simulink model "FMLibrary_v2_progress"  (R2016b)
settings: Solver=VariableStepAuto  StartTime=0.0  StopTime=10.0  RelTol=1e-3
undefined symbols (not defined in the file or in its folder): Lb, Lf, Lu, RobotStruct, sampleTime
libraries: simulink x24, FM_Library x10, VariousBlocksLibrary x10, FMLibrary_v2 x2, simulink_extras x2
(part 1 of 3)
settings Model: Creator=niekbeckers  LastModifiedBy=niekbeckers

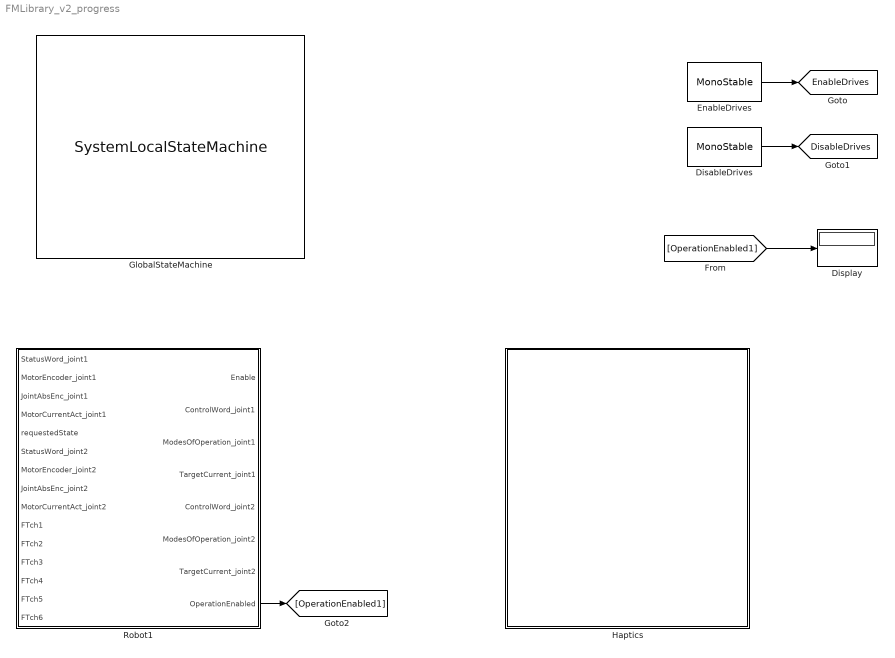
== system FMLibrary_v2_progress ==
  DisableDrives : FM_Library/MonoStable  Value=0  OutMin=[]  OutMax=[]  OutDataTypeStr=Inherit: Inherit from 'Constant value'
  Display : Display
  EnableDrives : FM_Library/MonoStable  Value=0  OutMin=[]  OutMax=[]  OutDataTypeStr=Inherit: Inherit from 'Constant value'
  GlobalStateMachine : FMLibrary_v2/StateMachineLocal/SystemLocalStateMachine
  Haptics : Subsystem
  Robot1 : Subsystem
  tag scope: DisableDrives=global, EnableDrives=global
  wires:
  DisableDrives/1 -> [DisableDrives]
  EnableDrives/1 -> [EnableDrives]
  Robot1/8(OperationEnabled) -> [OperationEnabled1]
  [OperationEnabled1] -> Display/1

== system FMLibrary_v2_progress/Haptics ==
  Bus Selector : BusSelector  OutputSignals=xOpSpace.x,xOpSpace.xdot
  tag scope: x_ref=global, xddot_ref=global, xdot_ref=global
  wires:
  [BusRobot1] -> Bus Selector/1

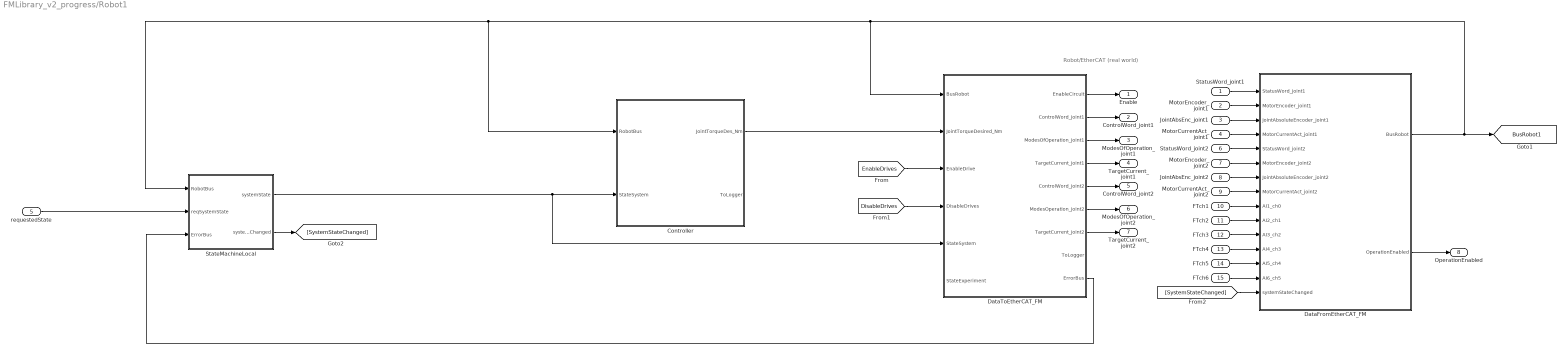
== system FMLibrary_v2_progress/Robot1 ==
  note: Robot/EtherCAT (real world)
  StatusWord_joint1 : Inport
  MotorEncoder_joint1 : Inport  Port=2
  JointAbsEnc_joint1 : Inport  Port=3
  MotorCurrentAct_joint1 : Inport  Port=4
  requestedState : Inport  Port=5
  StatusWord_joint2 : Inport  Port=6
  MotorEncoder_joint2 : Inport  Port=7
  JointAbsEnc_joint2 : Inport  Port=8
  MotorCurrentAct_joint2 : Inport  Port=9
  FTch1 : Inport  Port=10
  FTch2 : Inport  Port=11
  FTch3 : Inport  Port=12
  FTch4 : Inport  Port=13
  FTch5 : Inport  Port=14
  FTch6 : Inport  Port=15
  Controller : Subsystem  AncestorBlock=FMLibrary_v2/Controller
  DataFromEtherCAT_FM : Subsystem  AncestorBlock=FMLibrary_v2/DataFromEtherCAT_FM
  DataToEtherCAT_FM : Subsystem  AncestorBlock=FMLibrary_v2/DataToEtherCAT_FM
  StateMachineLocal : Subsystem  AncestorBlock=FMLibrary_v2/StateMachineLocal
  Enable : Outport
  ControlWord_joint1 : Outport  Port=2
  ModesOfOperation_joint1 : Outport  Port=3
  TargetCurrent_joint1 : Outport  Port=4
  ControlWord_joint2 : Outport  Port=5
  ModesOfOperation_joint2 : Outport  Port=6
  TargetCurrent_joint2 : Outport  Port=7
  OperationEnabled : Outport  Port=8
  tag scope: BusRobot1=global
  wires:
  DataFromEtherCAT_FM/2(OperationEnabled) -> OperationEnabled/1
  FTch3/1 -> DataFromEtherCAT_FM/11(AI3_ch2)
  FTch4/1 -> DataFromEtherCAT_FM/12(AI4_ch3)
  FTch6/1 -> DataFromEtherCAT_FM/14(AI6_ch5)
  StatusWord_joint2/1 -> DataFromEtherCAT_FM/5(StatusWord_joint2)
  StatusWord_joint1/1 -> DataFromEtherCAT_FM/1(StatusWord_joint1)
  DataToEtherCAT_FM/6(ModesOperation_joint2) -> ModesOfOperation_joint2/1
  DataToEtherCAT_FM/5(ControlWord_joint2) -> ControlWord_joint2/1
  MotorEncoder_joint1/1 -> DataFromEtherCAT_FM/2(MotorEncoder_joint1)
  JointAbsEnc_joint2/1 -> DataFromEtherCAT_FM/7("JointAbsoluteEncoder_joint2 ")
  FTch5/1 -> DataFromEtherCAT_FM/13(AI5_ch4)
  DataToEtherCAT_FM/4(TargetCurrent_joint1) -> TargetCurrent_joint1/1
  MotorCurrentAct_joint2/1 -> DataFromEtherCAT_FM/8(MotorCurrentAct_joint2)
  [EnableDrives] -> DataToEtherCAT_FM/3(EnableDrive)
  [DisableDrives] -> DataToEtherCAT_FM/4(DisableDrives)
  Controller/1(JointTorqueDes_Nm) -> DataToEtherCAT_FM/2(JointTorqueDesired_Nm)
  requestedState/1 -> StateMachineLocal/2(reqSystemState)
  DataFromEtherCAT_FM/1(BusRobot) -> [BusRobot1], DataToEtherCAT_FM/1(BusRobot), Controller/1(RobotBus), StateMachineLocal/1(RobotBus)
  DataToEtherCAT_FM/9(ErrorBus) -> StateMachineLocal/3(ErrorBus)
  [SystemStateChanged] -> DataFromEtherCAT_FM/15(systemStateChanged)
  StateMachineLocal/2(systemStateChanged) -> [SystemStateChanged]
  DataToEtherCAT_FM/2(ControlWord_joint1) -> ControlWord_joint1/1
  StateMachineLocal/1(systemState) -> DataToEtherCAT_FM/5(StateSystem), Controller/2(StateSystem)
  FTch1/1 -> DataFromEtherCAT_FM/9(AI1_ch0)
  DataToEtherCAT_FM/1(EnableCircuit) -> Enable/1
  DataToEtherCAT_FM/3(ModesOfOperation_joint1) -> ModesOfOperation_joint1/1
  JointAbsEnc_joint1/1 -> DataFromEtherCAT_FM/3(JointAbsoluteEncoder_joint1)
  MotorEncoder_joint2/1 -> DataFromEtherCAT_FM/6(MotorEncoder_joint2)
  MotorCurrentAct_joint1/1 -> DataFromEtherCAT_FM/4(MotorCurrentAct_joint1)
  FTch2/1 -> DataFromEtherCAT_FM/10(AI2_ch1)
  DataToEtherCAT_FM/7(TargetCurrent_joint2) -> TargetCurrent_joint2/1

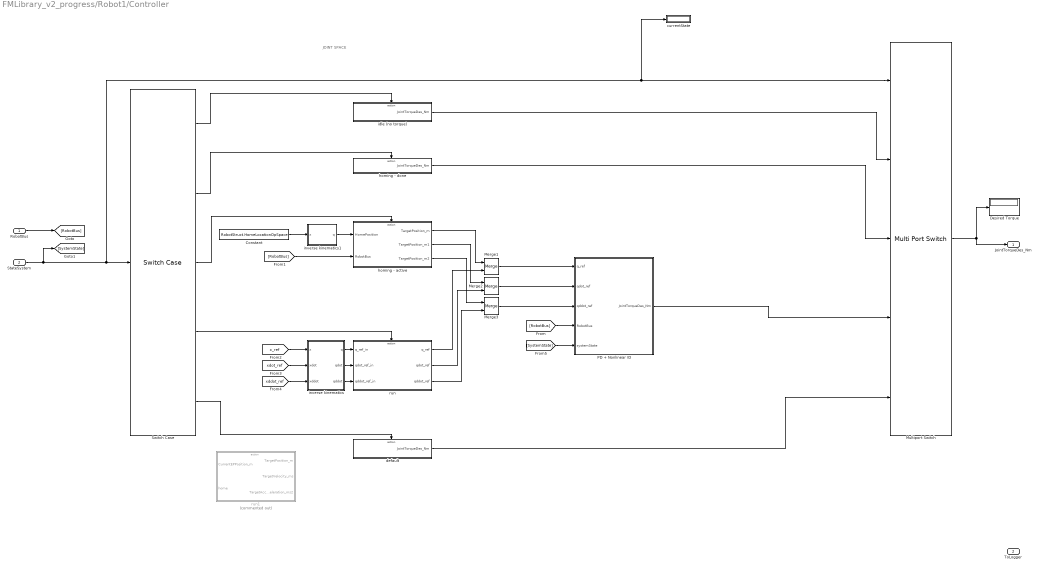
== system FMLibrary_v2_progress/Robot1/Controller ==
  note: JOINT SPACE
  RobotBus : Inport
  StateSystem : Inport  Port=2
  Constant : Constant  Value=RobotStruct.HomeLocationOpSpace
  Desired Torque : Display
  Merge1 : Merge  InitialOutput=[0;0]
  Merge2 : Merge  InitialOutput=[0;0]
  Merge3 : Merge  InitialOutput=[0;0]
  Multiport Switch : MultiPortSwitch  DataPortOrder=Specify indices  Inputs=4  DataPortIndices={[0,1,2,201,299,301],[399],[302,4]}  DataPortForDefault=Additional data port
  PD + Nonlinear ID : Subsystem
  Switch Case : SwitchCase  CaseConditions={[0,1,2,201,299,301],[399],[302],[4]}
  currentState : Display
  default : Subsystem  TreatAsAtomicUnit=on
  homing - active : Subsystem
  homing - done : Subsystem  TreatAsAtomicUnit=on
  idle (no torque) : Subsystem  TreatAsAtomicUnit=on
  inverse kinematics : MATLAB Function  TreatAsAtomicUnit=on
  inverse kinematics1 : MATLAB Function  TreatAsAtomicUnit=on
  run : Subsystem
  run1 : Subsystem  Commented=on
  JointTorqueDes_Nm : Outport
  ToLogger : Outport  Port=2
  wires:
  homing - active/3(TargetPosition_m2) -> Merge3/1
  homing - active/2(TargetPosition_m1) -> Merge2/1
  run/3(qddot_ref) -> Merge3/2
  run/2(qdot_ref) -> Merge2/2
  StateSystem/1 -> [SystemState], Switch Case/1, currentState/1, Multiport Switch/1
  run/1(q_ref) -> Merge1/2
  homing - active/1(TargetPosition_m) -> Merge1/1
  Switch Case/4 -> run/Action
  Multiport Switch/1 -> JointTorqueDes_Nm/1, Desired Torque/1
  Switch Case/5 -> default/Action
  default/1(JointTorqueDes_Nm) -> Multiport Switch/5
  Switch Case/1 -> idle (no torque)/Action
  Switch Case/3 -> homing - active/Action
  Switch Case/2 -> homing - done/Action
  idle (no torque)/1(JointTorqueDes_Nm) -> Multiport Switch/2
  homing - done/1(JointTorqueDes_Nm) -> Multiport Switch/3
  Merge1/1 -> PD + Nonlinear ID/1(q_ref)
  Merge2/1 -> PD + Nonlinear ID/2(qdot_ref)
  Merge3/1 -> PD + Nonlinear ID/3(qddot_ref)
  PD + Nonlinear ID/1(JointTorqueDes_Nm) -> Multiport Switch/4
  RobotBus/1 -> [RobotBus]
  [RobotBus] -> PD + Nonlinear ID/4(RobotBus)
  [RobotBus] -> homing - active/2(RobotBus)
  Constant/1 -> inverse kinematics1/1(x)
  inverse kinematics/1(q) -> run/1(q_ref_in)
  inverse kinematics/2(qdot) -> run/2(qdot_ref_in)
  inverse kinematics/3(qddot) -> run/3(qddot_ref_in)
  [x_ref] -> inverse kinematics/1(x)
  [xdot_ref] -> inverse kinematics/2(xdot)
  [xddot_ref] -> inverse kinematics/3(xddot)
  inverse kinematics1/1(q) -> homing - active/1(HomePosition)
  [SystemState] -> PD + Nonlinear ID/5(systemState)

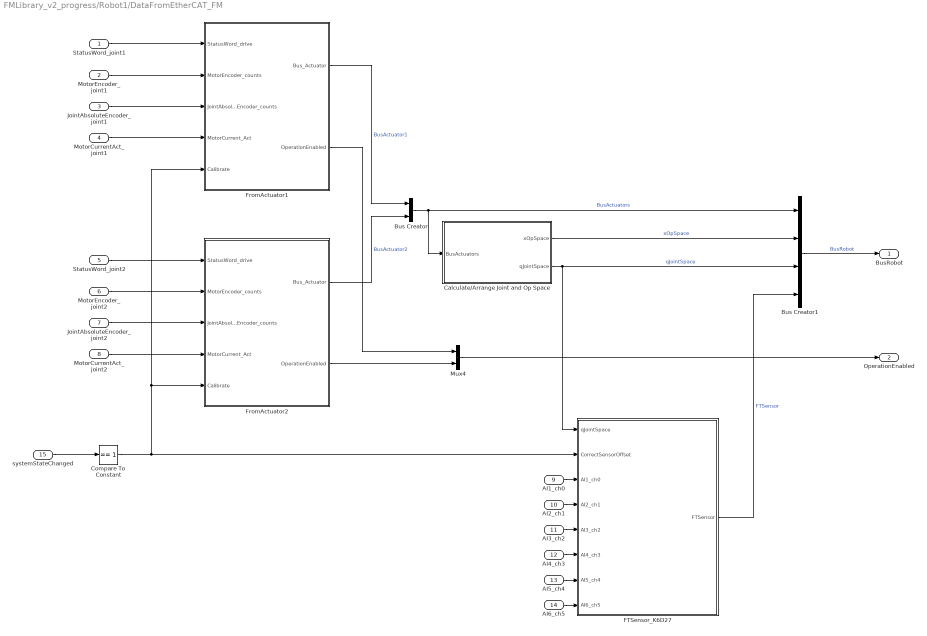
== system FMLibrary_v2_progress/Robot1/DataFromEtherCAT_FM ==
  StatusWord_joint1 : Inport
  MotorEncoder_joint1 : Inport  Port=2
  JointAbsoluteEncoder_joint1 : Inport  Port=3
  MotorCurrentAct_joint1 : Inport  Port=4
  StatusWord_joint2 : Inport  Port=5
  MotorEncoder_joint2 : Inport  Port=6
  "JointAbsoluteEncoder_joint2 " : Inport  Port=7
  MotorCurrentAct_joint2 : Inport  Port=8
  AI1_ch0 : Inport  Port=9  OutDataTypeStr=int16
  AI2_ch1 : Inport  Port=10  OutDataTypeStr=int16
  AI3_ch2 : Inport  Port=11  OutDataTypeStr=int16
  AI4_ch3 : Inport  Port=12  OutDataTypeStr=int16
  AI5_ch4 : Inport  Port=13  OutDataTypeStr=int16
  AI6_ch5 : Inport  Port=14  OutDataTypeStr=int16
  systemStateChanged : Inport  Port=15
  Bus Creator : BusCreator  Inputs=2
  Bus Creator1 : BusCreator  Inputs=4
  Calculate/Arrange Joint and Op Space : Subsystem
  Compare To Constant : simulink/Logic and Bit Operations/Compare To Constant  relop===  const=1  OutDataTypeStr=boolean
  FTSensor_K6D27 : Subsystem  mask{FTSensorStruct=RobotStruct.FTSensor}
      mask prompts: FTSensorStruct "Struct for force torque sensor"
  FromActuator1 : Subsystem  AncestorBlock=FMLibrary_v2/FromActuator1  mask{ActuatorStruct=RobotStruct.ActuatorStruct}
      mask prompts: ActuatorStruct "Actuator Struct"
  FromActuator2 : Subsystem  AncestorBlock=FMLibrary_v2/FromActuator1  mask{ActuatorStruct=RobotStruct.ActuatorStruct}
      mask prompts: ActuatorStruct "Actuator Struct"
  Mux4 : Mux  Inputs=2
  BusRobot : Outport
  OperationEnabled : Outport  Port=2
  wires:
  Compare To Constant/1 -> FTSensor_K6D27/2(CorrectSensorOffset), FromActuator1/5(Calibrate), FromActuator2/5(Calibrate)
  FTSensor_K6D27/1(FTSensor) -> Bus Creator1/4  "FTSensor"
  AI6_ch5/1 -> FTSensor_K6D27/8(AI6_ch5)
  AI5_ch4/1 -> FTSensor_K6D27/7(AI5_ch4)
  AI4_ch3/1 -> FTSensor_K6D27/6(AI4_ch3)
  AI3_ch2/1 -> FTSensor_K6D27/5(AI3_ch2)
  AI2_ch1/1 -> FTSensor_K6D27/4(AI2_ch1)
  AI1_ch0/1 -> FTSensor_K6D27/3(AI1_ch0)
  systemStateChanged/1 -> Compare To Constant/1
  Calculate/Arrange Joint and Op Space/2(qJointSpace) -> Bus Creator1/3, FTSensor_K6D27/1(qJointSpace)  "qJointSpace"
  Calculate/Arrange Joint and Op Space/1(xOpSpace) -> Bus Creator1/2  "xOpSpace"
  Bus Creator1/1 -> BusRobot/1  "BusRobot"
  Bus Creator/1 -> Bus Creator1/1, Calculate/Arrange Joint and Op Space/1(BusActuators)  "BusActuators"
  MotorCurrentAct_joint2/1 -> FromActuator2/4(MotorCurrent_Act)
  "JointAbsoluteEncoder_joint2 "/1 -> FromActuator2/3(JointAbsoluteEncoder_counts)
  StatusWord_joint2/1 -> FromActuator2/1(StatusWord_drive)
  MotorEncoder_joint2/1 -> FromActuator2/2(MotorEncoder_counts)
  MotorCurrentAct_joint1/1 -> FromActuator1/4(MotorCurrent_Act)
  JointAbsoluteEncoder_joint1/1 -> FromActuator1/3(JointAbsoluteEncoder_counts)
  StatusWord_joint1/1 -> FromActuator1/1(StatusWord_drive)
  MotorEncoder_joint1/1 -> FromActuator1/2(MotorEncoder_counts)
  FromActuator2/2(OperationEnabled) -> Mux4/2
  Mux4/1 -> OperationEnabled/1
  FromActuator1/2(OperationEnabled) -> Mux4/1
  FromActuator2/1(Bus_Actuator) -> Bus Creator/2  "BusActuator2"
  FromActuator1/1(Bus_Actuator) -> Bus Creator/1  "BusActuator1"

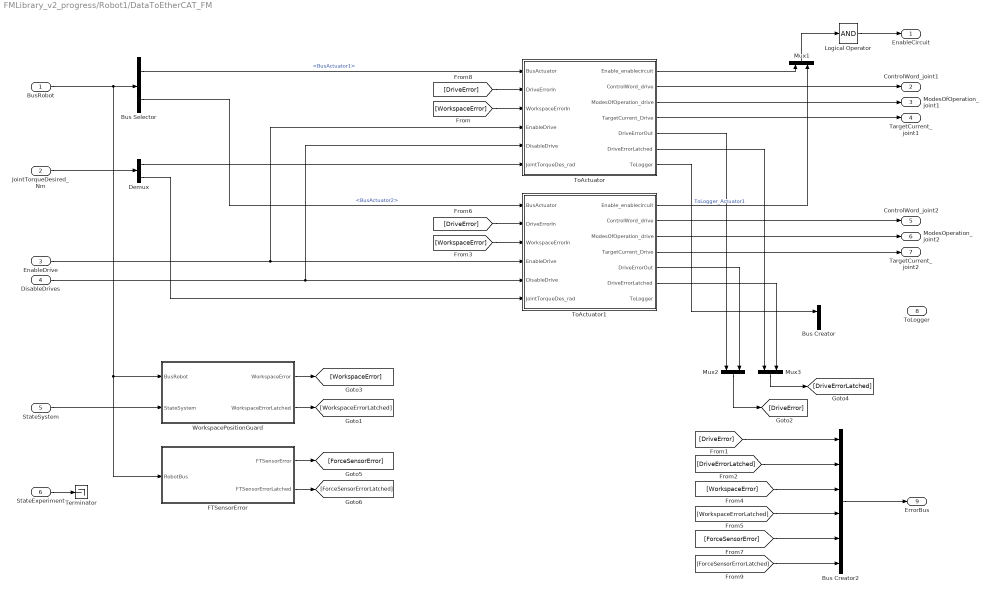
== system FMLibrary_v2_progress/Robot1/DataToEtherCAT_FM ==
  BusRobot : Inport
  JointTorqueDesired_Nm : Inport  Port=2
  EnableDrive : Inport  Port=3
  DisableDrives : Inport  Port=4
  StateSystem : Inport  Port=5
  StateExperiment : Inport  Port=6
  Bus Creator : BusCreator  Inputs=2
  Bus Creator2 : BusCreator  Inputs=6
  Bus Selector : BusSelector  OutputSignals=BusActuators.BusActuator1,BusActuators.BusActuator2
  Demux : Demux  Outputs=2
  FTSensorError : Subsystem
  Logical Operator : Logic  Inputs=1  AllPortsSameDT=off  OutDataTypeStr=boolean
  Mux1 : Mux  Inputs=2
  Mux2 : Mux  Inputs=2
  Mux3 : Mux  Inputs=2
  Terminator : Terminator
  ToActuator : Subsystem  AncestorBlock=FMLibrary_v2/ToActuator  mask{ActuatorStruct=RobotStruct.Actuator1}
      mask prompts: ActuatorStruct "Actuator Struct"
  ToActuator1 : Subsystem  AncestorBlock=FMLibrary_v2/ToActuator  mask{ActuatorStruct=RobotStruct.Actuator1}
      mask prompts: ActuatorStruct "Actuator Struct"
  WorkspacePositionGuard : Subsystem
  EnableCircuit : Outport
  ControlWord_joint1 : Outport  Port=2
  ModesOfOperation_joint1 : Outport  Port=3
  TargetCurrent_joint1 : Outport  Port=4
  ControlWord_joint2 : Outport  Port=5
  ModesOperation_joint2 : Outport  Port=6
  TargetCurrent_joint2 : Outport  Port=7
  ToLogger : Outport  Port=8
  ErrorBus : Outport  Port=9
  wires:
  StateExperiment/1 -> Terminator/1
  [ForceSensorErrorLatched] -> Bus Creator2/6
  [ForceSensorError] -> Bus Creator2/5
  FTSensorError/2(FTSensorErrorLatched) -> [ForceSensorErrorLatched]
  FTSensorError/1(FTSensorError) -> [ForceSensorError]
  StateSystem/1 -> WorkspacePositionGuard/2(StateSystem)
  [WorkspaceErrorLatched] -> Bus Creator2/4
  [WorkspaceError] -> Bus Creator2/3
  [DriveErrorLatched] -> Bus Creator2/2
  [DriveError] -> Bus Creator2/1
  Bus Creator2/1 -> ErrorBus/1
  Mux3/1 -> [DriveErrorLatched]
  [WorkspaceError] -> ToActuator1/3(WorkspaceErrorIn)
  [DriveError] -> ToActuator1/2(DriveErrorIn)
  EnableDrive/1 -> ToActuator1/4(EnableDrive), ToActuator/4(EnableDrive)
  DisableDrives/1 -> ToActuator1/5(DisableDrive), ToActuator/5(DisableDrive)
  [WorkspaceError] -> ToActuator/3(WorkspaceErrorIn)
  WorkspacePositionGuard/1(WorkspaceError) -> [WorkspaceError]
  WorkspacePositionGuard/2(WorkspaceErrorLatched) -> [WorkspaceErrorLatched]
  Bus Selector/1 -> ToActuator/1(BusActuator)  "<BusActuator1>"
  Bus Selector/2 -> ToActuator1/1(BusActuator)  "<BusActuator2>"
  BusRobot/1 -> Bus Selector/1, WorkspacePositionGuard/1(BusRobot), FTSensorError/1(RobotBus)
  Demux/1 -> ToActuator/6(JointTorqueDes_rad)
  JointTorqueDesired_Nm/1 -> Demux/1
  Demux/2 -> ToActuator1/6(JointTorqueDes_rad)
  Logical Operator/1 -> EnableCircuit/1
  ToActuator1/3(ModesOfOperation_drive) -> ModesOperation_joint2/1
  ToActuator1/4(TargetCurrent_Drive) -> TargetCurrent_joint2/1
  ToActuator/4(TargetCurrent_Drive) -> TargetCurrent_joint1/1
  ToActuator1/2(ControlWord_drive) -> ControlWord_joint2/1
  ToActuator/3(ModesOfOperation_drive) -> ModesOfOperation_joint1/1
  ToActuator/2(ControlWord_drive) -> ControlWord_joint1/1
  ToActuator1/1(Enable_enablecircuit) -> Mux1/2
  ToActuator/1(Enable_enablecircuit) -> Mux1/1
  Mux1/1 -> Logical Operator/1
  [DriveError] -> ToActuator/2(DriveErrorIn)
  ToActuator1/6(DriveErrorLatched) -> Mux3/2
  ToActuator/6(DriveErrorLatched) -> Mux3/1
  Mux2/1 -> [DriveError]
  ToActuator1/5(DriveErrorOut) -> Mux2/2
  ToActuator/5(DriveErrorOut) -> Mux2/1
  ToActuator/7(ToLogger) -> Bus Creator/1  "ToLogger_Actuator1"

== system FMLibrary_v2_progress/Robot1/StateMachineLocal ==
  note: Encode system state change - powers of 2 indicate which state change occurs.
  RobotBus : Inport
  reqSystemState : Inport  Port=2
  ErrorBus : Inport  Port=3
  Bus Selector : BusSelector  OutputSignals=xOpSpace.x,xOpSpace.xdot
  Constant : Constant  Value=RobotStruct.HomeLocationSize
  Constant1 : Constant  Value=RobotStruct.HomeLocationOpSpace
  Detect Change1 : simulink/Logic and Bit Operations/Detect Change  vinit=0  InputProcessing=Inherited  OutDataTypeStr=boolean
  Encode system state change : MATLAB Function  TreatAsAtomicUnit=on
  SystemLocalStateMachine : Stateflow chart  TreatAsAtomicUnit=on
  systemState : Outport
  systemStateChanged : Outport  Port=2
  wires:
  Bus Selector/2 -> SystemLocalStateMachine/4(xdot)  "<xdot>"
  Bus Selector/1 -> SystemLocalStateMachine/3(x)  "<x>"
  RobotBus/1 -> Bus Selector/1
  Constant1/1 -> SystemLocalStateMachine/5(HomePosition)
  Constant/1 -> SystemLocalStateMachine/6(homeLocationSize)
  Encode system state change/1(systemStateChanged) -> systemStateChanged/1
  Detect Change1/1 -> Encode system state change/1(stateChanged)
  ErrorBus/1 -> SystemLocalStateMachine/2(error)
  SystemLocalStateMachine/1(currentSystemState) -> Encode system state change/2(state), Detect Change1/1, systemState/1
  reqSystemState/1 -> SystemLocalStateMachine/1(reqSystemState)

== system FMLibrary_v2_progress/Robot1/Controller/PD + Nonlinear ID ==
  q_ref : Inport
  qdot_ref : Inport  Port=2
  qddot_ref : Inport  Port=3
  RobotBus : Inport  Port=4
  systemState : Inport  Port=5
  AFFC : Subsystem
  Bus Selector : BusSelector  OutputSignals=qJointSpace.q,qJointSpace.qdot
  DesiredTorque_PID : Display
  Gain : Gain
  Kd : Gain  Gain=0.1
  Kp : Gain  Gain=0.5
  Sum : Sum  Inputs=|+-
  Sum1 : Sum  Inputs=++|
  Sum2 : Sum  Inputs=|+-
  Sum3 : Sum  Inputs=|++
  p : Display
  JointTorqueDes_Nm : Outport
  wires:
  Bus Selector/2 -> Sum2/2  "<qdot>"
  Bus Selector/1 -> Sum/2  "<q>"
  q_ref/1 -> AFFC/1(q_ref), Sum/1
  Sum/1 -> Kp/1
  Sum3/1 -> AFFC/4(e), Sum1/2
  Kd/1 -> Sum3/2
  Kp/1 -> Sum3/1
  qdot_ref/1 -> AFFC/2(qdot_ref), Sum2/1
  Sum2/1 -> Kd/1
  Gain/1 -> Sum1/1
  Sum1/1 -> DesiredTorque_PID/1, JointTorqueDes_Nm/1
  RobotBus/1 -> Bus Selector/1
  qddot_ref/1 -> AFFC/3(qddot_ref)
  AFFC/1(p) -> p/1
  AFFC/2(tau_affc) -> Gain/1

== system FMLibrary_v2_progress/Robot1/Controller/default ==
  Action Port : ActionPort  InitializeStates=reset
  Constant3 : Constant  Value=[0;0]
  JointTorqueDes_Nm : Outport  InitialOutput=[0;0]
  wires:
  Constant3/1 -> JointTorqueDes_Nm/1

== system FMLibrary_v2_progress/Robot1/Controller/homing - active ==
  note: These blocks hold the first sample of the input
      | when the block is enabled (through the action port)
  HomePosition : Inport
  RobotBus : Inport  Port=2
  Action Port : ActionPort  InitializeStates=reset
  Bus Selector : BusSelector  OutputSignals=xOpSpace.x
  Constant1 : Constant
  Constant3 : Constant  Value=[0;0]
  Constant4 : Constant  Value=[0;0]
  Counter Free-Running : simulink/Sources/Counter Free-Running  NumBits=32  tsamp=-1
  CrossFade : VariousBlocksLibrary/Various/CrossFade
  Cycloid : VariousBlocksLibrary/Various/Cycloid
  Manual Switch : ManualSwitch  CurrentSetting=0
  Memory1 : Memory
  Rate Limiter : RateLimiter  RisingSlewLimit=0.2  FallingSlewLimit=-0.2  SampleTimeMode=inherited
  Switch : Switch  Threshold=1
  TargetPosition_m : Outport  InitialOutput=[0;0]
  TargetPosition_m1 : Outport  Port=2  InitialOutput=[0;0]
  TargetPosition_m2 : Outport  Port=3  InitialOutput=[0;0]
  wires:
  Constant4/1 -> TargetPosition_m2/1
  Constant3/1 -> TargetPosition_m1/1
  CrossFade/1 -> TargetPosition_m/1
  Manual Switch/1 -> CrossFade/1
  Memory1/1 -> Switch/1
  Counter Free-Running/1 -> Switch/2
  Switch/1 -> Manual Switch/1, Memory1/1
  Constant1/1 -> Rate Limiter/1
  Rate Limiter/1 -> Cycloid/1
  Cycloid/1 -> CrossFade/3
  HomePosition/1 -> CrossFade/2
  RobotBus/1 -> Bus Selector/1
  Bus Selector/1 -> Switch/3, Manual Switch/2  "<x>"

== system FMLibrary_v2_progress/Robot1/Controller/homing - done ==
  Action Port : ActionPort
  Constant : Constant  Value=[0;0]
  JointTorqueDes_Nm : Outport
  wires:
  Constant/1 -> JointTorqueDes_Nm/1

== system FMLibrary_v2_progress/Robot1/Controller/idle (no torque) ==
  Action Port : ActionPort  InitializeStates=reset
  Constant3 : Constant  Value=[0;0]
  JointTorqueDes_Nm : Outport
  wires:
  Constant3/1 -> JointTorqueDes_Nm/1

== system FMLibrary_v2_progress/Robot1/Controller/run ==
  q_ref_in : Inport
  qdot_ref_in : Inport  Port=2
  qddot_ref_in : Inport  Port=3
  Action Port : ActionPort  InitializeStates=reset
  q_ref : Outport
  qdot_ref : Outport  Port=2
  qddot_ref : Outport  Port=3
  wires:
  q_ref_in/1 -> q_ref/1
  qddot_ref_in/1 -> qddot_ref/1
  qdot_ref_in/1 -> qdot_ref/1

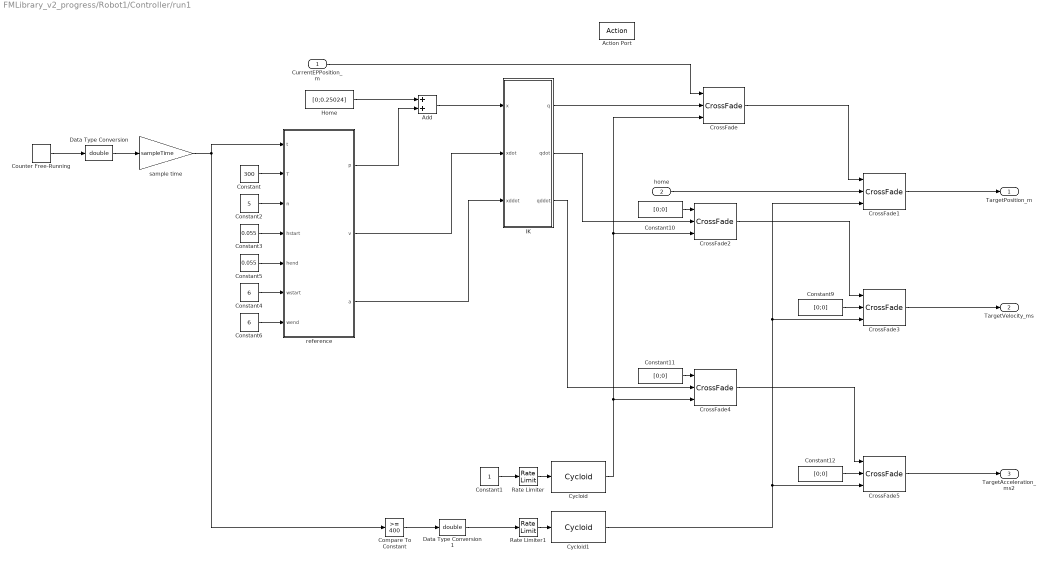
== system FMLibrary_v2_progress/Robot1/Controller/run1 ==
  CurrentEPPosition_m : Inport
  home : Inport  Port=2
  Action Port : ActionPort  InitializeStates=reset
  Add : Sum
  Compare To Constant : simulink/Logic and Bit Operations/Compare To Constant  relop=>=  const=400  OutDataTypeStr=boolean
  Constant : Constant  Value=300
  Constant1 : Constant
  Constant{9..12} (4 alike) : Constant  Value=[0;0]
  Constant2 : Constant  Value=5
  Constant3 : Constant  Value=0.055
  Constant4 : Constant  Value=6
  Constant5 : Constant  Value=0.055
  Constant6 : Constant  Value=6
  Counter Free-Running : simulink/Sources/Counter Free-Running  NumBits=32  tsamp=-1
  CrossFade{,1..5} (6 alike) : VariousBlocksLibrary/Various/CrossFade
  Cycloid : VariousBlocksLibrary/Various/Cycloid
  Cycloid1 : VariousBlocksLibrary/Various/Cycloid
  Data Type Conversion : DataTypeConversion  OutDataTypeStr=double
  Data Type Conversion1 : DataTypeConversion  OutDataTypeStr=double
  "Home " : Constant  Value=[0;0.25024]
  IK : MATLAB Function  TreatAsAtomicUnit=on
  Rate Limiter : RateLimiter  RisingSlewLimit=0.25  FallingSlewLimit=-0.15  SampleTimeMode=inherited
  Rate Limiter1 : RateLimiter  RisingSlewLimit=0.2  FallingSlewLimit=-0.2  SampleTimeMode=inherited
  reference : MATLAB Function  TreatAsAtomicUnit=on
  sample time : Gain  Gain=sampleTime
  TargetPosition_m : Outport
  TargetVelocity_ms : Outport  Port=2
  TargetAcceleration_ms2 : Outport  Port=3
  wires:
  Data Type Conversion1/1 -> Rate Limiter1/1
  IK/3(qddot) -> CrossFade4/2
  IK/1(q) -> CrossFade/2
  IK/2(qdot) -> CrossFade2/2
  "Home "/1 -> Add/1
  Add/1 -> IK/1(x)
  reference/1(p) -> Add/2
  reference/2(v) -> IK/2(xdot)
  reference/3(a) -> IK/3(xddot)
  Constant4/1 -> reference/6(wstart)
  Constant6/1 -> reference/7(wend)
  Constant3/1 -> reference/4(hstart)
  Constant5/1 -> reference/5(hend)
  Constant2/1 -> reference/3(n)
  Constant/1 -> reference/2(T)
  sample time/1 -> reference/1(t), Compare To Constant/1
  Counter Free-Running/1 -> Data Type Conversion/1
  Data Type Conversion/1 -> sample time/1
  CrossFade5/1 -> TargetAcceleration_ms2/1
  Constant11/1 -> CrossFade4/1
  Constant12/1 -> CrossFade5/2
  CrossFade4/1 -> CrossFade5/1
  Constant10/1 -> CrossFade2/1
  Constant9/1 -> CrossFade3/2
  CrossFade2/1 -> CrossFade3/1
  CrossFade3/1 -> TargetVelocity_ms/1
  Cycloid1/1 -> CrossFade1/3, CrossFade3/3, CrossFade5/3
  Rate Limiter1/1 -> Cycloid1/1
  Compare To Constant/1 -> Data Type Conversion1/1
  home/1 -> CrossFade1/2
  CrossFade/1 -> CrossFade1/1
  CrossFade1/1 -> TargetPosition_m/1
  CurrentEPPosition_m/1 -> CrossFade/1
  Rate Limiter/1 -> Cycloid/1
  Constant1/1 -> Rate Limiter/1
  Cycloid/1 -> CrossFade4/3, CrossFade/3, CrossFade2/3

== system FMLibrary_v2_progress/Robot1/DataFromEtherCAT_FM/Calculate//Arrange Joint and Op Space ==
  note: Here all angles of the parallel mechanism are calculated
      | based on the endpoint position, though this may still lead to incorrect
      | estimations of the internal angles (e.g. it is possible that on of the elbows
      | has gone through a singular position already). So perhaps I should also include
      | a different way of calculating the internal angles
  BusActuators : Inport
  Bus Creator1 : BusCreator  Inputs=3
  Bus Creator2 : BusCreator  Inputs=3
  Bus Selector : BusSelector  OutputSignals=BusActuator1.JointPosition_rad,BusActuator2.JointPosition_rad  OutputAsBus=on
  Bus Selector1 : BusSelector  OutputSignals=BusActuator1.JointVelocity_rads,BusActuator2.JointVelocity_rads  OutputAsBus=on
  Bus Selector2 : BusSelector  OutputSignals=BusActuator1.JointPosition_rad,BusActuator2.JointPosition_rad,BusActuator1.JointVelocity_rads,BusActuator2.JointVelocity_rads
  Ground : Ground
  IK all joints : MATLAB Function  TreatAsAtomicUnit=on
  Mux : Mux  Inputs=2
  Mux1 : Mux  Inputs=2
  Terminator1 : Terminator
  Terminator2 : Terminator
  forward kinematics : Subsystem
  xOpSpace : Outport
  qJointSpace : Outport  Port=2
  wires:
  IK all joints/1(q_all) -> Bus Creator2/3  "qall"
  Mux1/1 -> Bus Creator2/2  "qdot"
  Bus Selector2/4 -> Mux1/2  "<JointVelocity_rads>"
  Bus Selector2/3 -> Mux1/1  "<JointVelocity_rads>"
  Bus Selector2/2 -> Mux/2  "<JointPosition_rad>"
  Bus Selector2/1 -> Mux/1  "<JointPosition_rad>"
  Mux/1 -> Bus Creator2/1  "q"
  BusActuators/1 -> Bus Selector/1, Bus Selector2/1, Bus Selector1/1
  Bus Creator2/1 -> qJointSpace/1  "JointSpace"
  Ground/1 -> forward kinematics/3(JointAcceleration_rads2)
  Bus Selector1/1 -> forward kinematics/2(JointVelocity_rads)
  forward kinematics/4(J) -> Bus Creator1/3  "jacobian"
  Bus Creator1/1 -> xOpSpace/1  "OpSpace"
  forward kinematics/1(x) -> Bus Creator1/1, IK all joints/1(x)  "x"
  Bus Selector/1 -> forward kinematics/1(JointPosition_rad)
  forward kinematics/2(xdot) -> Bus Creator1/2  "xdot"
  forward kinematics/3(xddot) -> Terminator1/1
  forward kinematics/5(Jdot) -> Terminator2/1

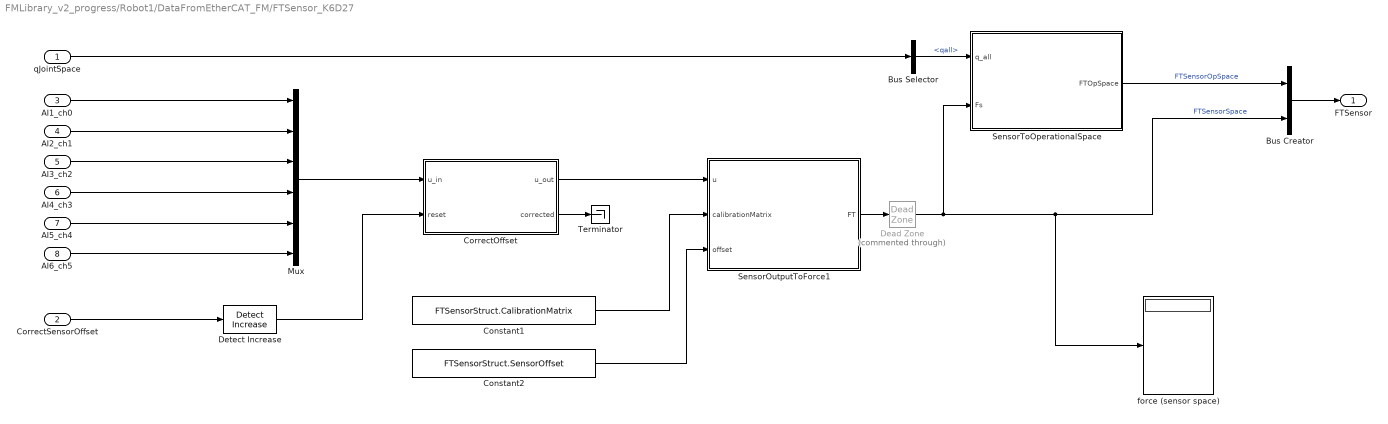
== system FMLibrary_v2_progress/Robot1/DataFromEtherCAT_FM/FTSensor_K6D27 ==
  qJointSpace : Inport
  CorrectSensorOffset : Inport  Port=2
  AI1_ch0 : Inport  Port=3  OutDataTypeStr=int16
  AI2_ch1 : Inport  Port=4  OutDataTypeStr=int16
  AI3_ch2 : Inport  Port=5  OutDataTypeStr=int16
  AI4_ch3 : Inport  Port=6  OutDataTypeStr=int16
  AI5_ch4 : Inport  Port=7  OutDataTypeStr=int16
  AI6_ch5 : Inport  Port=8  OutDataTypeStr=int16
  Bus Creator : BusCreator  Inputs=2
  Bus Selector : BusSelector  OutputSignals=qall
  Constant1 : Constant  Value=FTSensorStruct.CalibrationMatrix
  Constant2 : Constant  Value=FTSensorStruct.SensorOffset
  CorrectOffset : MATLAB Function  TreatAsAtomicUnit=on
  Dead Zone : DeadZone  Commented=through  LowerValue=-0.05  UpperValue=0.05  SaturateOnIntegerOverflow=on
  Detect Increase : simulink/Logic and Bit Operations/Detect Increase  vinit=0.0  InputProcessing=Inherited  OutDataTypeStr=boolean
  Mux : Mux  Inputs=6
  SensorOutputToForce1 : MATLAB Function  TreatAsAtomicUnit=on
  SensorToOperationalSpace : MATLAB Function  TreatAsAtomicUnit=on
  Terminator : Terminator
  force (sensor space) : Display
  FTSensor : Outport
  wires:
  SensorToOperationalSpace/1(FTOpSpace) -> Bus Creator/1  "FTSensorOpSpace"
  Bus Creator/1 -> FTSensor/1
  Constant2/1 -> SensorOutputToForce1/3(offset)
  Constant1/1 -> SensorOutputToForce1/2(calibrationMatrix)
  Dead Zone/1 -> SensorToOperationalSpace/2(Fs), force (sensor space)/1, Bus Creator/2  "FTSensorSpace"
  CorrectOffset/2(corrected) -> Terminator/1
  AI3_ch2/1 -> Mux/3
  AI4_ch3/1 -> Mux/4
  AI5_ch4/1 -> Mux/5
  AI6_ch5/1 -> Mux/6
  Bus Selector/1 -> SensorToOperationalSpace/1(q_all)  "<qall>"
  SensorOutputToForce1/1(FT) -> Dead Zone/1
  Detect Increase/1 -> CorrectOffset/2(reset)
  CorrectSensorOffset/1 -> Detect Increase/1
  Mux/1 -> CorrectOffset/1(u_in)
  CorrectOffset/1(u_out) -> SensorOutputToForce1/1(u)
  AI1_ch0/1 -> Mux/1
  AI2_ch1/1 -> Mux/2
  qJointSpace/1 -> Bus Selector/1

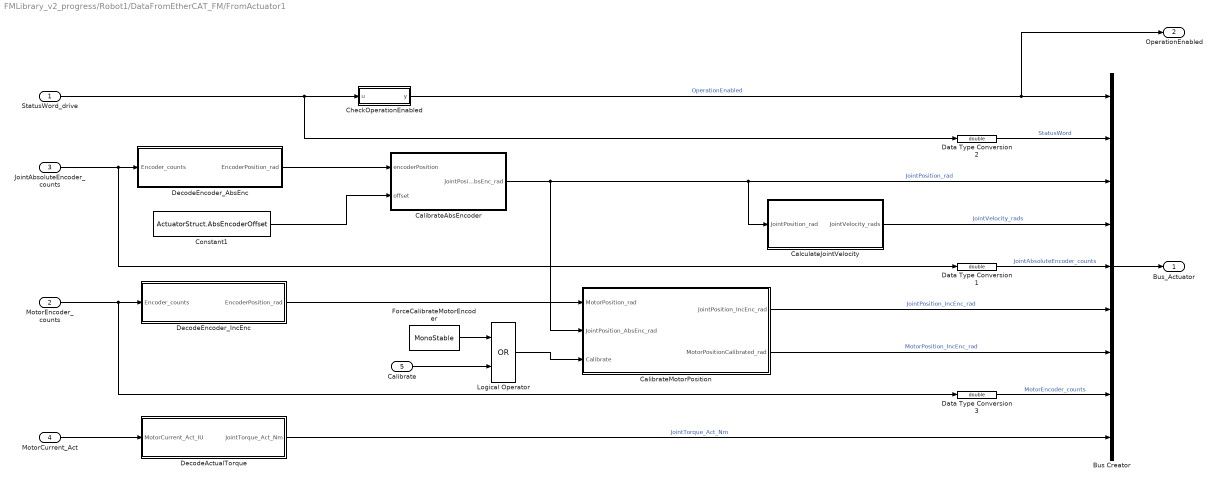
== system FMLibrary_v2_progress/Robot1/DataFromEtherCAT_FM/FromActuator1 ==
  StatusWord_drive : Inport
  MotorEncoder_counts : Inport  Port=2
  JointAbsoluteEncoder_counts : Inport  Port=3
  MotorCurrent_Act : Inport  Port=4
  Calibrate : Inport  Port=5
  Bus Creator : BusCreator  Inputs=9
  CalculateJointVelocity : Subsystem
  CalibrateAbsEncoder : MATLAB Function  TreatAsAtomicUnit=on
  "CalibrateMotorPosition    " : MATLAB Function  TreatAsAtomicUnit=on  mask{gearboxRatio=ActuatorStruct.transmissionRatio}
      mask prompts: gearboxRatio "Transmission ratio (e.g. -8) [-]"
  CheckOperationEnabled : MATLAB Function  TreatAsAtomicUnit=on
  Constant1 : Constant  Value=ActuatorStruct.AbsEncoderOffset
  Data Type Conversion1 : DataTypeConversion  OutDataTypeStr=double
  Data Type Conversion2 : DataTypeConversion  OutDataTypeStr=double
  Data Type Conversion3 : DataTypeConversion  OutDataTypeStr=double
  DecodeActualTorque : MATLAB Function  TreatAsAtomicUnit=on  mask(DecodeActualTorque){transmissionRatio=ActuatorStruct.transmissionRatio, motorTorqueConstant=ActuatorStruct.motorTorqueConstant, drivePeakCurrent=ActuatorStruct.drivePeakCurrent}
      mask prompts: transmissionRatio "Transmission ratio (e.g. -8) [-]"; motorTorqueConstant "Motor torque constant [Nm/A]"; drivePeakCurrent "Motor drive peak current Ipeak [A]"
      mask help:
      | Decode Actual Torque value returned from the actuator (motor drive and motor) to torque on the joint (after transmission).
      |
      | Note: due to the way the transmission is set up and the positive motor axis (clockwise is positive as seen from the motor front), there is no need to account for sign change in motor torque or encoder position.
  DecodeEncoder_AbsEnc : MATLAB Function  TreatAsAtomicUnit=on  mask(DecodeEncoder){EncoderCounts_rev=ActuatorStruct.JointAbsoluteEncoderCounts_rev}
      mask prompts: EncoderCounts_rev "Motor encoder increments per revolution (e.g., 8192)"
      mask help: Decode the encoder counts to encoder position in radians
  DecodeEncoder_IncEnc : MATLAB Function  TreatAsAtomicUnit=on  mask(DecodeEncoder){EncoderCounts_rev=ActuatorStruct.MotorEncoderCounts_rev}
      mask prompts: EncoderCounts_rev "Motor encoder increments per revolution (e.g., 8192)"
      mask help: Decode the encoder counts to encoder position in radians
  ForceCalibrateMotorEncoder : FM_Library/MonoStable  Value=0  OutMin=[]  OutMax=[]  OutDataTypeStr=Inherit: Inherit from 'Constant value'
  Logical Operator : Logic  Operator=OR  AllPortsSameDT=off  OutDataTypeStr=boolean
  Bus_Actuator : Outport
  OperationEnabled : Outport  Port=2
  wires:
  ForceCalibrateMotorEncoder/1 -> Logical Operator/1
  Constant1/1 -> CalibrateAbsEncoder/2(offset)
  Logical Operator/1 -> "CalibrateMotorPosition    "/3(Calibrate)
  Bus Creator/1 -> Bus_Actuator/1
  Data Type Conversion3/1 -> Bus Creator/8  "MotorEncoder_counts"
  MotorEncoder_counts/1 -> Data Type Conversion3/1, DecodeEncoder_IncEnc/1(Encoder_counts)
  CalibrateAbsEncoder/1(JointPosition_AbsEnc_rad) -> Bus Creator/3, CalculateJointVelocity/1(JointPosition_rad), "CalibrateMotorPosition    "/2(JointPosition_AbsEnc_rad)  "JointPosition_rad"
  Data Type Conversion2/1 -> Bus Creator/2  "StatusWord"
  Data Type Conversion1/1 -> Bus Creator/5  "JointAbsoluteEncoder_counts"
  "CalibrateMotorPosition    "/1(JointPosition_IncEnc_rad) -> Bus Creator/6  "JointPosition_IncEnc_rad"
  JointAbsoluteEncoder_counts/1 -> DecodeEncoder_AbsEnc/1(Encoder_counts), Data Type Conversion1/1
  CheckOperationEnabled/1(y) -> Bus Creator/1, OperationEnabled/1  "OperationEnabled"
  MotorCurrent_Act/1 -> DecodeActualTorque/1(MotorCurrent_Act_IU)
  DecodeEncoder_IncEnc/1(EncoderPosition_rad) -> "CalibrateMotorPosition    "/1(MotorPosition_rad)
  StatusWord_drive/1 -> CheckOperationEnabled/1(u), Data Type Conversion2/1
  DecodeActualTorque/1(JointTorque_Act_Nm) -> Bus Creator/9  "JointTorque_Act_Nm"
  "CalibrateMotorPosition    "/2(MotorPositionCalibrated_rad) -> Bus Creator/7  "MotorPosition_IncEnc_rad"
  DecodeEncoder_AbsEnc/1(EncoderPosition_rad) -> CalibrateAbsEncoder/1(encoderPosition)
  CalculateJointVelocity/1(JointVelocity_rads) -> Bus Creator/4  "JointVelocity_rads"
  Calibrate/1 -> Logical Operator/2

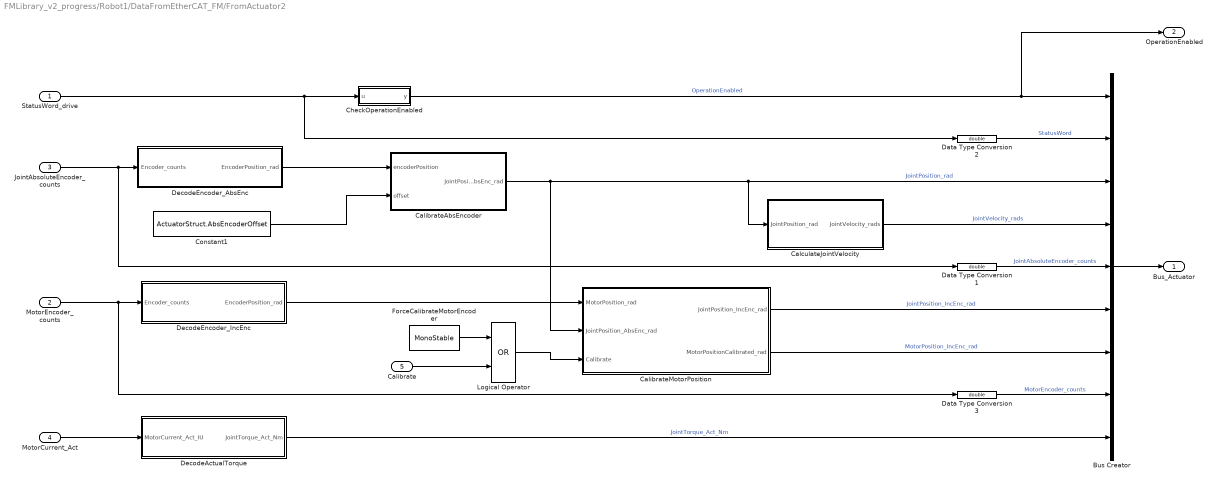
== system FMLibrary_v2_progress/Robot1/DataFromEtherCAT_FM/FromActuator2 ==
  StatusWord_drive : Inport
  MotorEncoder_counts : Inport  Port=2
  JointAbsoluteEncoder_counts : Inport  Port=3
  MotorCurrent_Act : Inport  Port=4
  Calibrate : Inport  Port=5
  Bus Creator : BusCreator  Inputs=9
  CalculateJointVelocity : Subsystem
  CalibrateAbsEncoder : MATLAB Function  TreatAsAtomicUnit=on
  "CalibrateMotorPosition    " : MATLAB Function  TreatAsAtomicUnit=on  mask{gearboxRatio=ActuatorStruct.transmissionRatio}
      mask prompts: gearboxRatio "Transmission ratio (e.g. -8) [-]"
  CheckOperationEnabled : MATLAB Function  TreatAsAtomicUnit=on
  Constant1 : Constant  Value=ActuatorStruct.AbsEncoderOffset
  Data Type Conversion1 : DataTypeConversion  OutDataTypeStr=double
  Data Type Conversion2 : DataTypeConversion  OutDataTypeStr=double
  Data Type Conversion3 : DataTypeConversion  OutDataTypeStr=double
  DecodeActualTorque : MATLAB Function  TreatAsAtomicUnit=on  mask(DecodeActualTorque){transmissionRatio=ActuatorStruct.transmissionRatio, motorTorqueConstant=ActuatorStruct.motorTorqueConstant, drivePeakCurrent=ActuatorStruct.drivePeakCurrent}
      mask prompts: transmissionRatio "Transmission ratio (e.g. -8) [-]"; motorTorqueConstant "Motor torque constant [Nm/A]"; drivePeakCurrent "Motor drive peak current Ipeak [A]"
      mask help:
      | Decode Actual Torque value returned from the actuator (motor drive and motor) to torque on the joint (after transmission).
      |
      | Note: due to the way the transmission is set up and the positive motor axis (clockwise is positive as seen from the motor front), there is no need to account for sign change in motor torque or encoder position.
  DecodeEncoder_AbsEnc : MATLAB Function  TreatAsAtomicUnit=on  mask(DecodeEncoder){EncoderCounts_rev=ActuatorStruct.JointAbsoluteEncoderCounts_rev}
      mask prompts: EncoderCounts_rev "Motor encoder increments per revolution (e.g., 8192)"
      mask help: Decode the encoder counts to encoder position in radians
  DecodeEncoder_IncEnc : MATLAB Function  TreatAsAtomicUnit=on  mask(DecodeEncoder){EncoderCounts_rev=ActuatorStruct.MotorEncoderCounts_rev}
      mask prompts: EncoderCounts_rev "Motor encoder increments per revolution (e.g., 8192)"
      mask help: Decode the encoder counts to encoder position in radians
  ForceCalibrateMotorEncoder : FM_Library/MonoStable  Value=0  OutMin=[]  OutMax=[]  OutDataTypeStr=Inherit: Inherit from 'Constant value'
  Logical Operator : Logic  Operator=OR  AllPortsSameDT=off  OutDataTypeStr=boolean
  Bus_Actuator : Outport
  OperationEnabled : Outport  Port=2
  wires:
  ForceCalibrateMotorEncoder/1 -> Logical Operator/1
  Constant1/1 -> CalibrateAbsEncoder/2(offset)
  Logical Operator/1 -> "CalibrateMotorPosition    "/3(Calibrate)
  Bus Creator/1 -> Bus_Actuator/1
  Data Type Conversion3/1 -> Bus Creator/8  "MotorEncoder_counts"
  MotorEncoder_counts/1 -> Data Type Conversion3/1, DecodeEncoder_IncEnc/1(Encoder_counts)
  CalibrateAbsEncoder/1(JointPosition_AbsEnc_rad) -> Bus Creator/3, CalculateJointVelocity/1(JointPosition_rad), "CalibrateMotorPosition    "/2(JointPosition_AbsEnc_rad)  "JointPosition_rad"
  Data Type Conversion2/1 -> Bus Creator/2  "StatusWord"
  Data Type Conversion1/1 -> Bus Creator/5  "JointAbsoluteEncoder_counts"
  "CalibrateMotorPosition    "/1(JointPosition_IncEnc_rad) -> Bus Creator/6  "JointPosition_IncEnc_rad"
  JointAbsoluteEncoder_counts/1 -> DecodeEncoder_AbsEnc/1(Encoder_counts), Data Type Conversion1/1
  CheckOperationEnabled/1(y) -> Bus Creator/1, OperationEnabled/1  "OperationEnabled"
  MotorCurrent_Act/1 -> DecodeActualTorque/1(MotorCurrent_Act_IU)
  DecodeEncoder_IncEnc/1(EncoderPosition_rad) -> "CalibrateMotorPosition    "/1(MotorPosition_rad)
  StatusWord_drive/1 -> CheckOperationEnabled/1(u), Data Type Conversion2/1
  DecodeActualTorque/1(JointTorque_Act_Nm) -> Bus Creator/9  "JointTorque_Act_Nm"
  "CalibrateMotorPosition    "/2(MotorPositionCalibrated_rad) -> Bus Creator/7  "MotorPosition_IncEnc_rad"
  DecodeEncoder_AbsEnc/1(EncoderPosition_rad) -> CalibrateAbsEncoder/1(encoderPosition)
  CalculateJointVelocity/1(JointVelocity_rads) -> Bus Creator/4  "JointVelocity_rads"
  Calibrate/1 -> Logical Operator/2

== system FMLibrary_v2_progress/Robot1/DataToEtherCAT_FM/FTSensorError ==
  RobotBus : Inport
  AvoidAlgebraicLoop : Memory
  Bus Selector1 : BusSelector  OutputSignals=FTSensor.FTSensorSpace
  Constant : Constant  Value=RobotStruct.MaxAllowableForcesTorqueSensor
  CreateSingleErrorValue : FMLibrary_v2/DataToEtherCAT_FM/WorkspacePositionGuard/CreateSingleErrorValue
  Detect Change : simulink/Logic and Bit Operations/Detect Change  vinit=0  InputProcessing=Inherited  OutDataTypeStr=boolean
  FTSensorLastError : Display
  LatchRising : FM_Library/LatchRising  ic=0
  MATLAB Function : MATLAB Function  TreatAsAtomicUnit=on
  ShowFTSensorErrorLatched : Display
  FTSensorError : Outport
  FTSensorErrorLatched : Outport  Port=2
  wires:
  Constant/1 -> MATLAB Function/2(MaxForcesTorques)
  MATLAB Function/1(e) -> FTSensorLastError/1, CreateSingleErrorValue/1
  Bus Selector1/1 -> MATLAB Function/1(ForcesTorques)  "<FTSensorSpace>"
  RobotBus/1 -> Bus Selector1/1
  CreateSingleErrorValue/1 -> AvoidAlgebraicLoop/1
  LatchRising/1 -> ShowFTSensorErrorLatched/1, FTSensorErrorLatched/1
  AvoidAlgebraicLoop/1 -> LatchRising/1, Detect Change/1, FTSensorError/1
  Detect Change/1 -> LatchRising/Trigger

== system FMLibrary_v2_progress/Robot1/DataToEtherCAT_FM/ToActuator ==
  note: The Latched version keeps the most recent value from when the motor was on; in other words, the reason why the motor turned off.
  note: The UseActuator block can be used to enable or disable the actuator altogether.
  BusActuator : Inport
  DriveErrorIn : Inport  Port=2
  WorkspaceErrorIn : Inport  Port=3
  EnableDrive : Inport  Port=4
  DisableDrive : Inport  Port=5
  JointTorqueDes_rad : Inport  Port=6
  AppendToBus : Subsystem
  DriveEnableLogic : Subsystem
  EncodeDesiredTorque : MATLAB Function  TreatAsAtomicUnit=on  mask(EncodeDesiredTorque){transmissionRatio=ActuatorStruct.transmissionRatio, motorTorqueConstant=ActuatorStruct.motorTorqueConstant, drivePeakCurrent=ActuatorStruct.drivePeakCurrent}
      mask prompts: transmissionRatio "Transmission ratio (e.g. -8) [-]"; motorTorqueConstant "Motor torque constant [Nm/A]"; drivePeakCurrent "Motor drive peak current [A]"
      mask help:
      | Encode desired torque at the joint to torque to be produced by the motor.
      |
      | Note: due to the way the transmission is set up and the positive motor axis (clockwise is positive as seen from the motor front), there is no need to account for sign change in motor torque or encoder position.
  PreventAlgebraicLoop : Memory
  TorqueLimit_Nm : Constant  Value=ActuatorStruct.TorqueLimit_Nm
  TorqueLimiter : FM_Library/TorqueLimiter
  UseActuator : Constant  OutDataTypeStr=double
      settings: OpenFcn=|
      | b = get_param(gcb,'value');
      | if (strcmp(b,'1')),
      |   set_param (gcb,'value','0');
      | else
      |   set_param(gcb,'value','1');
      | end;
  Enable_enablecircuit : Outport
  ControlWord_drive : Outport  Port=2
  ModesOfOperation_drive : Outport  Port=3
  TargetCurrent_Drive : Outport  Port=4
  DriveErrorOut : Outport  Port=5
  DriveErrorLatched : Outport  Port=6
  ToLogger : Outport  Port=7
  wires:
  WorkspaceErrorIn/1 -> DriveEnableLogic/5(WorkspaceErrorIn)
  DriveEnableLogic/1(Enable_enablecircuit) -> Enable_enablecircuit/1
  JointTorqueDes_rad/1 -> AppendToBus/3(DesiredTorque), TorqueLimiter/2
  TorqueLimiter/1 -> DriveEnableLogic/7(TorqueGuardMax)
  TorqueLimiter/2 -> AppendToBus/4(DesiredTorqueLimited), EncodeDesiredTorque/1(JointTorque_Des_Nm)
  DriveEnableLogic/5(DriveErrorOutLatched) -> DriveErrorLatched/1
  TorqueLimit_Nm/1 -> TorqueLimiter/1
  DriveEnableLogic/3(ModesOfOperation_drive) -> ModesOfOperation_drive/1
  DriveEnableLogic/2(ControlWord_drive) -> ControlWord_drive/1
  EncodeDesiredTorque/1(MotorTorque_Des_IU) -> TargetCurrent_Drive/1
  BusActuator/1 -> DriveEnableLogic/6(BusActuators), AppendToBus/1(Bus_in)
  EnableDrive/1 -> DriveEnableLogic/1(EnableDrive)
  DisableDrive/1 -> DriveEnableLogic/2(DisableDrive)
  DriveEnableLogic/4(DriveErrorOut) -> AppendToBus/2(DriveError), PreventAlgebraicLoop/1
  DriveErrorIn/1 -> DriveEnableLogic/4(DriveErrorIn)
  PreventAlgebraicLoop/1 -> DriveErrorOut/1
  AppendToBus/1(Bus_out) -> ToLogger/1
  UseActuator/1 -> DriveEnableLogic/3(UseActuator)

== system FMLibrary_v2_progress/Robot1/DataToEtherCAT_FM/ToActuator1 ==
  note: The Latched version keeps the most recent value from when the motor was on; in other words, the reason why the motor turned off.
  note: The UseActuator block can be used to enable or disable the actuator altogether.
  BusActuator : Inport
  DriveErrorIn : Inport  Port=2
  WorkspaceErrorIn : Inport  Port=3
  EnableDrive : Inport  Port=4
  DisableDrive : Inport  Port=5
  JointTorqueDes_rad : Inport  Port=6
  AppendToBus : Subsystem
  DriveEnableLogic : Subsystem
  EncodeDesiredTorque : MATLAB Function  TreatAsAtomicUnit=on  mask(EncodeDesiredTorque){transmissionRatio=ActuatorStruct.transmissionRatio, motorTorqueConstant=ActuatorStruct.motorTorqueConstant, drivePeakCurrent=ActuatorStruct.drivePeakCurrent}
      mask prompts: transmissionRatio "Transmission ratio (e.g. -8) [-]"; motorTorqueConstant "Motor torque constant [Nm/A]"; drivePeakCurrent "Motor drive peak current [A]"
      mask help:
      | Encode desired torque at the joint to torque to be produced by the motor.
      |
      | Note: due to the way the transmission is set up and the positive motor axis (clockwise is positive as seen from the motor front), there is no need to account for sign change in motor torque or encoder position.
  PreventAlgebraicLoop : Memory
  TorqueLimit_Nm : Constant  Value=ActuatorStruct.TorqueLimit_Nm
  TorqueLimiter : FM_Library/TorqueLimiter
  UseActuator : Constant  OutDataTypeStr=double
      settings: OpenFcn=|
      | b = get_param(gcb,'value');
      | if (strcmp(b,'1')),
      |   set_param (gcb,'value','0');
      | else
      |   set_param(gcb,'value','1');
      | end;
  Enable_enablecircuit : Outport
  ControlWord_drive : Outport  Port=2
  ModesOfOperation_drive : Outport  Port=3
  TargetCurrent_Drive : Outport  Port=4
  DriveErrorOut : Outport  Port=5
  DriveErrorLatched : Outport  Port=6
  ToLogger : Outport  Port=7
  wires:
  WorkspaceErrorIn/1 -> DriveEnableLogic/5(WorkspaceErrorIn)
  DriveEnableLogic/1(Enable_enablecircuit) -> Enable_enablecircuit/1
  JointTorqueDes_rad/1 -> AppendToBus/3(DesiredTorque), TorqueLimiter/2
  TorqueLimiter/1 -> DriveEnableLogic/7(TorqueGuardMax)
  TorqueLimiter/2 -> AppendToBus/4(DesiredTorqueLimited), EncodeDesiredTorque/1(JointTorque_Des_Nm)
  DriveEnableLogic/5(DriveErrorOutLatched) -> DriveErrorLatched/1
  TorqueLimit_Nm/1 -> TorqueLimiter/1
  DriveEnableLogic/3(ModesOfOperation_drive) -> ModesOfOperation_drive/1
  DriveEnableLogic/2(ControlWord_drive) -> ControlWord_drive/1
  EncodeDesiredTorque/1(MotorTorque_Des_IU) -> TargetCurrent_Drive/1
  BusActuator/1 -> DriveEnableLogic/6(BusActuators), AppendToBus/1(Bus_in)
  EnableDrive/1 -> DriveEnableLogic/1(EnableDrive)
  DisableDrive/1 -> DriveEnableLogic/2(DisableDrive)
  DriveEnableLogic/4(DriveErrorOut) -> AppendToBus/2(DriveError), PreventAlgebraicLoop/1
  DriveErrorIn/1 -> DriveEnableLogic/4(DriveErrorIn)
  PreventAlgebraicLoop/1 -> DriveErrorOut/1
  AppendToBus/1(Bus_out) -> ToLogger/1
  UseActuator/1 -> DriveEnableLogic/3(UseActuator)

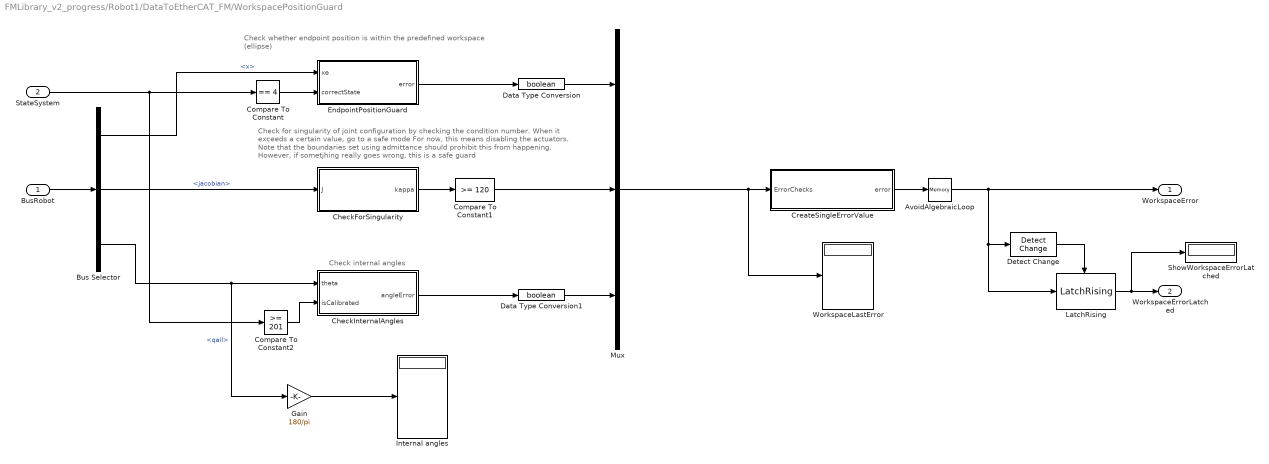
== system FMLibrary_v2_progress/Robot1/DataToEtherCAT_FM/WorkspacePositionGuard ==
  note: Check for singularity of joint configuration by checking
      | the condition number. When it exceeds a certain value, go to a safe mode
      | For now, this means disabling the actuators.
      | Note that the boundaries set using admittance should prohibit this from happening.
      | However, if sometjhing really goes wrong, this is a safe guard
  note: Check whether endpoint position is within the predefined workspace
      | (ellipse)
  note: Check internal angles
  BusRobot : Inport
  StateSystem : Inport  Port=2
  AvoidAlgebraicLoop : Memory
  Bus Selector : BusSelector  OutputSignals=xOpSpace.x,xOpSpace.jacobian,qJointSpace.qall
  CheckForSingularity : MATLAB Function  TreatAsAtomicUnit=on
  CheckInternalAngles : MATLAB Function  TreatAsAtomicUnit=on
  Compare To Constant : simulink/Logic and Bit Operations/Compare To Constant  relop===  const=4  OutDataTypeStr=boolean
  Compare To Constant1 : simulink/Logic and Bit Operations/Compare To Constant  relop=>=  const=120  OutDataTypeStr=boolean
  Compare To Constant2 : simulink/Logic and Bit Operations/Compare To Constant  relop=>=  const=201  OutDataTypeStr=boolean
  CreateSingleErrorValue : Subsystem
  Data Type Conversion : DataTypeConversion  OutDataTypeStr=boolean
  Data Type Conversion1 : DataTypeConversion  OutDataTypeStr=boolean
  Detect Change : simulink/Logic and Bit Operations/Detect Change  vinit=0  InputProcessing=Inherited  OutDataTypeStr=boolean
  EndpointPositionGuard : MATLAB Function  TreatAsAtomicUnit=on
  Gain : Gain  Gain=180/pi
  Internal angles : Display
  LatchRising : FM_Library/LatchRising  ic=0
  Mux : Mux  Inputs=3
  ShowWorkspaceErrorLatched : Display
  WorkspaceLastError : Display
  WorkspaceError : Outport
  WorkspaceErrorLatched : Outport  Port=2
  wires:
  StateSystem/1 -> Compare To Constant/1, Compare To Constant2/1
  Bus Selector/2 -> CheckForSingularity/1(J)  "<jacobian>"
  Gain/1 -> Internal angles/1
  Compare To Constant2/1 -> CheckInternalAngles/2(isCalibrated)
  Compare To Constant/1 -> EndpointPositionGuard/2(correctState)
  AvoidAlgebraicLoop/1 -> WorkspaceError/1, LatchRising/1, Detect Change/1
  Detect Change/1 -> LatchRising/Trigger
  CreateSingleErrorValue/1(error) -> AvoidAlgebraicLoop/1
  Data Type Conversion1/1 -> Mux/3
  Data Type Conversion/1 -> Mux/1
  Compare To Constant1/1 -> Mux/2
  LatchRising/1 -> WorkspaceErrorLatched/1, ShowWorkspaceErrorLatched/1
  CheckInternalAngles/1(angleError) -> Data Type Conversion1/1
  Bus Selector/3 -> CheckInternalAngles/1(theta), Gain/1  "<qall>"
  Bus Selector/1 -> EndpointPositionGuard/1(xe)  "<x>"
  BusRobot/1 -> Bus Selector/1
  EndpointPositionGuard/1(error) -> Data Type Conversion/1
  Mux/1 -> CreateSingleErrorValue/1(ErrorChecks), WorkspaceLastError/1
  CheckForSingularity/1(kappa) -> Compare To Constant1/1

== system FMLibrary_v2_progress/Robot1/Controller/PD + Nonlinear ID/AFFC ==
  q_ref : Inport
  qdot_ref : Inport  Port=2
  qddot_ref : Inport  Port=3
  e : Inport  Port=4
  AFFC : MATLAB Function  TreatAsAtomicUnit=on
  Counter Free-Running : simulink/Sources/Counter Free-Running  NumBits=32  tsamp=-1
  Data Type Conversion : DataTypeConversion  OutDataTypeStr=double
  Learning factors : Constant  Value=[2e-5;1e-2;1e-3;1e-3]
  sample time : Gain  Gain=sampleTime
  p : Outport
  tau_affc : Outport  Port=2
  wires:
  Learning factors/1 -> AFFC/6(w)
  Data Type Conversion/1 -> sample time/1
  sample time/1 -> AFFC/1(t)
  Counter Free-Running/1 -> Data Type Conversion/1
  AFFC/1(p) -> p/1
  AFFC/2(tau) -> tau_affc/1
  q_ref/1 -> AFFC/2(q)
  qdot_ref/1 -> AFFC/3(qdot)
  qddot_ref/1 -> AFFC/4(qddot)
  e/1 -> AFFC/5(e)

== system FMLibrary_v2_progress/Robot1/DataFromEtherCAT_FM/Calculate//Arrange Joint and Op Space/forward kinematics ==
  JointPosition_rad : Inport  PortDimensions=[2 1]
  JointVelocity_rads : Inport  Port=2  PortDimensions=[2 1]
  JointAcceleration_rads2 : Inport  Port=3  PortDimensions=[2 1]
  Je : MATLAB Function  TreatAsAtomicUnit=on
  Jedot : MATLAB Function  TreatAsAtomicUnit=on
  Product : Product  Multiplication=Matrix(*)
  calculate xddot : MATLAB Function  TreatAsAtomicUnit=on
  forward kinematics : MATLAB Function  TreatAsAtomicUnit=on
  x : Outport
  xdot : Outport  Port=2
  xddot : Outport  Port=3
  J : Outport  Port=4
  Jdot : Outport  Port=5
  wires:
  JointAcceleration_rads2/1 -> calculate xddot/1(qddot)
  calculate xddot/1(xddot) -> xddot/1
  forward kinematics/1(x) -> x/1
  Product/1 -> xdot/1
  Jedot/1(Jedot) -> Jdot/1, calculate xddot/4(Jdot)
  JointVelocity_rads/1 -> Jedot/2(qdot), Product/2, calculate xddot/2(qdot)
  Je/1(Je) -> J/1, Product/1, calculate xddot/3(J)
  JointPosition_rad/1 -> Je/1(q), Jedot/1(q), forward kinematics/1(q)

== system FMLibrary_v2_progress/Robot1/DataFromEtherCAT_FM/FromActuator1/CalculateJointVelocity ==
  JointPosition_rad : Inport
  Discrete Derivative : simulink/Discrete/Discrete Derivative  Commented=on  gainval=1.0  ICPrevScaledInput=0.0  InputProcessing=Inherited  OutMin=[]  OutMax=[]  OutDataType=fixdt(1, 16)  OutScaling=2^-10  DoSatur=off
  FOAW : MATLAB Function  TreatAsAtomicUnit=on
  Filter1 : FM_Library/FilterFourthOrder/Filter1  Commented=on  sampleTime=sampleTime
  Omega1 : Constant  Commented=on  Value=2*pi*100  OutDataTypeStr=double
  encoder noise : Constant  Value=ActuatorStruct.FOAWNoiseLevel
  JointVelocity_rads : Outport
  wires:
  encoder noise/1 -> FOAW/2(noise)
  FOAW/1(xdot) -> JointVelocity_rads/1
  Omega1/1 -> Filter1/2
  Discrete Derivative/1 -> Filter1/1
  Filter1/1 -> ?
  JointPosition_rad/1 -> FOAW/1(x)

== system FMLibrary_v2_progress/Robot1/DataFromEtherCAT_FM/FromActuator2/CalculateJointVelocity ==
  JointPosition_rad : Inport
  Discrete Derivative : simulink/Discrete/Discrete Derivative  Commented=on  gainval=1.0  ICPrevScaledInput=0.0  InputProcessing=Inherited  OutMin=[]  OutMax=[]  OutDataType=fixdt(1, 16)  OutScaling=2^-10  DoSatur=off
  FOAW : MATLAB Function  TreatAsAtomicUnit=on
  Filter1 : FM_Library/FilterFourthOrder/Filter1  Commented=on  sampleTime=sampleTime
  Omega1 : Constant  Commented=on  Value=2*pi*100  OutDataTypeStr=double
  encoder noise : Constant  Value=ActuatorStruct.FOAWNoiseLevel
  JointVelocity_rads : Outport
  wires:
  encoder noise/1 -> FOAW/2(noise)
  FOAW/1(xdot) -> JointVelocity_rads/1
  Omega1/1 -> Filter1/2
  Discrete Derivative/1 -> Filter1/1
  Filter1/1 -> ?
  JointPosition_rad/1 -> FOAW/1(x)

== system FMLibrary_v2_progress/Robot1/DataToEtherCAT_FM/ToActuator/AppendToBus ==
  Bus_in : Inport
  DriveError : Inport  Port=2
  DesiredTorque : Inport  Port=3
  DesiredTorqueLimited : Inport  Port=4
  Bus Creator : BusCreator  Inputs=12
  Bus Selector2 : BusSelector  OutputSignals=OperationEnabled,StatusWord,JointPosition_rad,JointVelocity_rads,MotorEncoder_counts,MotorPosition_IncEnc_rad,JointPosition_IncEnc_rad,JointAbsoluteEncoder_counts,JointTorque_Act_Nm
  Data Type Conversion : DataTypeConversion  OutDataTypeStr=double
  Bus_out : Outport
  wires:
  Bus Selector2/9 -> Bus Creator/9  "<JointTorque_Act_Nm>"
  Bus Creator/1 -> Bus_out/1
  Bus_in/1 -> Bus Selector2/1
  DriveError/1 -> Data Type Conversion/1
  Data Type Conversion/1 -> Bus Creator/12  "DriveError"
  DesiredTorque/1 -> Bus Creator/10  "DesiredTorque_Nm"
  DesiredTorqueLimited/1 -> Bus Creator/11  "DesiredTorqueLimited_Nm"
  Bus Selector2/1 -> Bus Creator/1  "<OperationEnabled>"
  Bus Selector2/2 -> Bus Creator/2  "<StatusWord>"
  Bus Selector2/3 -> Bus Creator/3  "<JointPosition_rad>"
  Bus Selector2/4 -> Bus Creator/4  "<JointVelocity_rads>"
  Bus Selector2/5 -> Bus Creator/5  "<MotorEncoder_counts>"
  Bus Selector2/7 -> Bus Creator/7  "<JointPosition_IncEnc_rad>"
  Bus Selector2/8 -> Bus Creator/8  "<JointAbsoluteEncoder_counts>"
  Bus Selector2/6 -> Bus Creator/6  "<MotorPosition_IncEnc_rad>"
